simulink model "otro"  (R2018a)
settings: Solver=VariableStepAuto  StartTime=0.0  StopTime=84  RelTol=1e-3
settings Model: Creator=Dell  LastModifiedBy=Dell

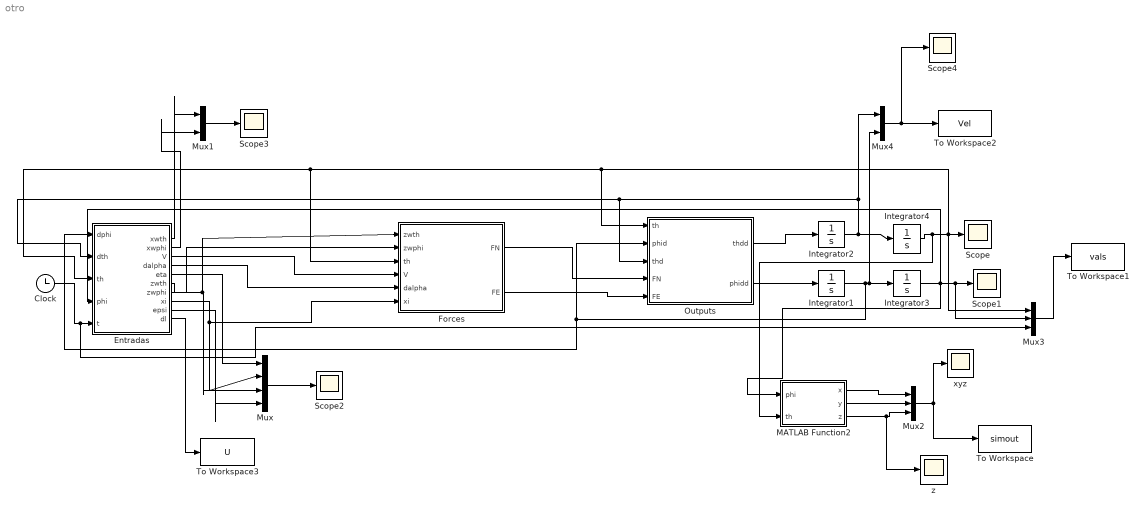
== system otro ==
  Clock : Clock
  Entradas : MATLAB Function  TreatAsAtomicUnit=on
  Forces : MATLAB Function  TreatAsAtomicUnit=on
  Integrator1 : Integrator  LowerSaturationLimit=0
  Integrator2 : Integrator
  Integrator3 : Integrator
  Integrator4 : Integrator  LimitOutput=on  LowerSaturationLimit=-0.000001
  MATLAB Function2 : MATLAB Function  TreatAsAtomicUnit=on
  Mux : Mux
  Mux1 : Mux  Inputs=2
  Mux2 : Mux  Inputs=3
  Mux3 : Mux  Inputs=3
  Mux4 : Mux  Inputs=2
  Outputs : MATLAB Function  TreatAsAtomicUnit=on
  Scope{,1..4} (5 alike) : Scope
  To Workspace : ToWorkspace  VariableName=simout  SampleTime=-1
  To Workspace1 : ToWorkspace  VariableName=vals  SampleTime=-1
  To Workspace2 : ToWorkspace  VariableName=Vel  SampleTime=-1
  To Workspace3 : ToWorkspace  VariableName=U  SampleTime=-1
  xyz : Scope
  z : Scope
  wires:
  Forces/1(FN) -> Outputs/4(FN)
  Forces/2(FE) -> Outputs/5(FE)
  Entradas/4(dalpha) -> Forces/5(dalpha)
  Entradas/3(V) -> Forces/4(V)
  Clock/1 -> Mux3/3, Entradas/5(t)
  Outputs/2(phidd) -> Integrator1/1
  Outputs/1(thdd) -> Integrator2/1
  Integrator1/1 -> Outputs/2(phid), Entradas/1(dphi), Mux4/2, Integrator3/1
  Integrator2/1 -> Mux4/1, Outputs/3(thd), Entradas/2(dth), Integrator4/1
  Integrator3/1 -> MATLAB Function2/1(phi), Mux3/2, Scope1/1, Entradas/4(phi)
  Integrator4/1 -> MATLAB Function2/2(th), Mux3/1, Scope/1, Outputs/1(th), Entradas/3(th), Forces/3(th)
  Entradas/5(eta) -> Mux/1
  Entradas/8(xi) -> Forces/6(xi), Mux/2
  Entradas/6(zwth) -> Forces/1(zwth), Mux/3
  Entradas/9(epsi) -> Mux/4
  Mux/1 -> Scope2/1
  Entradas/7(zwphi) -> Forces/2(zwphi)
  Entradas/1(xwth) -> Mux1/1
  Entradas/2(xwphi) -> Mux1/2
  Mux1/1 -> Scope3/1
  Mux2/1 -> xyz/1, To Workspace/1
  MATLAB Function2/3(z) -> z/1, Mux2/3
  MATLAB Function2/1(x) -> Mux2/1
  MATLAB Function2/2(y) -> Mux2/2
  Mux3/1 -> To Workspace1/1
  Mux4/1 -> Scope4/1, To Workspace2/1
  Entradas/10(dl) -> To Workspace3/1

== matlab function otro/Forces ==
  data: zwth input; zwphi input; th input; V input; dalpha input; xi input; FN output; FE output
function [FN,FE] = fcn(zwth,zwphi,th,V,dalpha,xi)

m= 0.256; %7 ;%0.256 kg;
g= 9.81; 
CD= 0.0316;%0.75;%0.15 ; %.75;              % generara errores almover los coeficientes
CL=   0.1354; %1;%0.85;  %1;        %  siguiente simulación agregare  los parametros de CD y CL  obtenidos mediante el software 
CDl= 0.002;
%er=[0;0;1];

Al= pi*(0.03/2^2);
% hacer una grafica como la de Higth altitude   
Rho= 1.2; % kg/m^3
A= 2.2;  % m^2 %  30 miguel 
%Wa=[0;0;0];


Faerth= (CL*A*Rho*V^2)*zwth-(Rho*(CD)*V^2*A*(cos(xi)*cos(dalpha))); 
FGth=  -m*g*cos(th)  ;                                    %[-m*g*cos(th);0;m*g*sin(th)];
Faerphi= (CL*A*Rho*V^2)*zwphi-(Rho*(CD)*V^2*A*(sin(xi)*cos(dalpha))); 
FGphi=  0 ;                                    %[-m*g*cos(th);0;m*g*sin(th)];
%F= FG+Faer;
FN= FGth+Faerth ;                 %dot(F,eN);
FE=    Faerphi+FGphi;                %dot(F,eL);

== matlab function otro/Outputs ==
  data: th input; thdd output; phid input; thd input; FN input; FE input; phidd output
function [thdd,phidd]= fcn(th,phid,thd,FN,FE)
m= 0.256 ;     %7; miguel
% 0.256 %yo en gramos ;
r=35;

%Fg= [-m*g*cos(th);0;m*g*sin(th)];
%F0= [0;0;0];
%Fth= dot(FN,en)+.3;%dot(Fg,en);
%Fphi= dot(FE,ele)+.2; %dot(Fg,ele);
%Fr= 0;
thdd=FN/(2*m*r)-sin(th)*cos(th)*phid^2;  % modificar  no va rm  entre todos despejar de esto    
phidd= (FE/(r*m*cos(th)))+2*tan(th)*thd*phid;  % checar con fuerza aparente esta es deacuerdo a Miguel  lo otro no

== matlab function otro/Entradas ==
  data: dphi input; dth input; th input; phi input; xwth output; xwphi output; V output; dalpha output; eta output; zwth output; zwphi output; xi output; t input; epsi output; dl output
function [xwth,xwphi,V,dalpha,eta,zwth,zwphi,xi,epsi,dl] = fcn(dphi,dth,th,phi,t)
Wx= 7;  
%yo  6 
r=35;
dr=0;
dl=0;
if t<=75
     dl= 0; 
end
  if t >= 75 &&  t <= 78
  dl= 0;
 
  end
   if t >= 78 &&  t <= 180
  dl= 0;
   end
  


%dl=0;%sin(t*.22)*.65;  %sin(t*.22)*.65 % sin entrada  de esta classe igual a 0 se comporta igual al sistema de dos stage sin valores reales de zw
%k=sin(t*.10)*.65;
ws= 2.4; %2.5;
% er=[0;0;1];
% eL=[0;1;0];
% eN=[1;0;0];
epsi= asin(dl/ws);
%W0= [Wx;0;0];         
wlt=[-Wx*cos(phi)*sin(th);-Wx*sin(phi);-Wx*cos(phi)*cos(th)];
Vk= [r*dth;r*dphi*cos(th);0];
Wa= wlt-Vk;
V= norm(Wa);
xi= atan2((Wx*sin(phi)+dphi*r*cos(th)),(dth*r+Wx*cos(phi)*sin(th))); %checar segundo termino si esta mal no es phip es thp
dalpha= asin((Wx*cos(phi)*cos(th))/((Wx*sin(phi)+dphi*r*cos(th))^2+(r*dth+Wx*cos(phi)*sin(th))^2+(dr+Wx*cos(phi)*cos(th))^2)^(1/2)); %si es + y checar ecu

eta= asin(tan(dalpha)*tan(epsi)); % ten'ia tan de xi y es tan(Dalpha)

xwth= -cos(xi)*cos(dalpha);
xwphi=  -sin(xi)*cos(dalpha);
zwth= cos(xi)*cos(epsi)*cos(eta)*sin(dalpha)-sin(xi)*cos(epsi)*sin(eta)*sin(dalpha)-sin(xi)*sin(epsi)*cos(dalpha);  
zwphi=  sin(xi)*cos(epsi)*cos(eta)*sin(dalpha)+cos(xi)*(cos(epsi)*sin(eta)*sin(dalpha)+sin(epsi)*cos(dalpha));        

%plot3(simout(:,1),simout(:,2),simout(:,3)) plot 3d
%grid

== matlab function otro/MATLAB Function2 ==
  data: x output; phi input; y output; th input; z output
function [x,y,z]= fcn(phi,th)
r=35;
x= r*cos(phi)*cos(th);
y= r*sin(phi)*cos(th);
z= r*sin(th);
